simulink model "ev"  (R2021a)
settings: Solver=ode4  StartTime=0  StopTime=1082  FixedStep=sim_dt  RelTol=1e-3
model workspace (MAT data in the model file):
  T_eff_bp = [-270; -210; -150; -90; -30; 30; 90; 150; 210; 270]
  T_eff_bp_2 = [-270; -210; -150; -90; -30; 30; 90; 150; 210; 270]
  losses_table = [108927.107777 7820.2782368 7820.17609997 7820.2782368 7820.2782368 7820.2782368 7820.2782368 7820.26172359 7820.2782368 9345.38006027 108927.107777 7820.2782368 ... (100 elements, 10x10)]
  losses_table_2 = [108927.107777 7820.2782368 7820.17609997 7820.2782368 7820.2782368 7820.2782368 7820.2782368 7820.26172359 7820.2782368 9345.38006027 108927.107777 7820.2782368 ... (100 elements, 10x10)]
  w_eff_bp = [0; 888.888888889; 1777.77777778; 2666.66666667; 3555.55555556; 4444.44444444; 5333.33333333; 6222.22222222; 7111.11111111; 8000]
  w_eff_bp_2 = [0; 888.888888889; 1777.77777778; 2666.66666667; 3555.55555556; 4444.44444444; 5333.33333333; 6222.22222222; 7111.11111111; 8000]
undefined symbols (not defined in the file): Af, alpha, Bt, C, C_fa, C_free, C_sa_bat, C_sa_uc, Cd, Cmax, Continuous, Crr, DoD, effi, etaFD, etaG, FD, G, gear, Iucmax, m, M1m, M2m, Max, npar, npar_free, npara, nparf, nparfa, nparsa_bat, nparsa_UC, nser, nser_free, nserfa, nsersa_bat, nsersa_UC, Qbat, regenmax, Ri_BP, RL, ro, Rsc, Rsc_A, Rsc_F, Rsc_sa_bat, Rsc_sa_uc, rw, sim_dt, SOC_BP, SoCbatmax, SoCbatmin, SoCucmax, SoCucmin, speed, torque, VinBat, Voc_BP, Vuc, Vuc_fa, Vuc_free ... (+2)
libraries: autolibshared x41, simulink x26, autolibdcdc x13, autolibdatasheetbattery x7, autolibmappedmotor x6, fl_lib x3, nesl_utility x3, spsSupercapacitorLib x3, pid_lib x1
(part 3 of 18)

== system ev/Drive cycle power demand/Controller. Actual motor torque ==
  motor angular speed : Inport
  wheel torque : Inport  Port=2
  Power_motor_out : Inport  Port=3
  1-D Lookup Table : Lookup_n-D  NumberOfTableDimensions=1  BreakpointsForDimension1=Continuous(:,1)  Table=Continuous(:,2)  InternalRulePriority=Speed  RndMeth=Simplest  InputSameDT=on
  1-D Lookup Table2 : Lookup_n-D  NumberOfTableDimensions=1  BreakpointsForDimension1=Continuous(:,1)  Table=-Continuous(:,2)  InternalRulePriority=Speed  RndMeth=Simplest  InputSameDT=on
  Constant : Constant
  Delay : Delay  DelayLength=1  InitialCondition=1
  Delay1 : Delay  DelayLength=1  InitialCondition=0
  Equal : RelationalOperator  Operator===  OutDataTypeStr=boolean  RndMeth=Simplest
  Gain1 : Gain  Gain=30/pi
  Gain2 : Gain  Gain=30/pi
  Gain3 : Gain  Gain=30/pi
  GreaterThanOrEqual : RelationalOperator  OutDataTypeStr=boolean  RndMeth=Simplest
  MATLAB Function : MATLAB Function  TreatAsAtomicUnit=on
  Mux1 : Mux  Inputs=3
  Mux2 : Mux  Inputs=2
  Mux3 : Mux  Inputs=2
  Product : Product
  Product1 : Product
  Product2 : Product
  Saturation Dynamic : simulink/Discontinuities/Saturation Dynamic  OutMin=[]  OutMax=[]  OutDataTypeStr=Inherit: Same as second input  OutDataType=fixdt(1, 16)  OutScaling=2^-10  DoSatur=off
  Scope{6..14} (9 alike) : Scope
  Tapped Delay : simulink/Discrete/Tapped Delay  vinit=1  samptime=-1  NumDelays=30  DelayOrder=Oldest  includeCurrent=off
  To Workspace : ToWorkspace  VariableName=n_mtr  SaveFormat=Structure With Time  SampleTime=-1
  To Workspace1 : ToWorkspace  VariableName=com  SaveFormat=Structure With Time  SampleTime=-1
  To Workspace2 : ToWorkspace  VariableName=zz_motor_trq  SaveFormat=Structure With Time  SampleTime=-1
  To Workspace3 : ToWorkspace  VariableName=zz_motor_speed  SaveFormat=Structure With Time  SampleTime=-1
  To Workspace4 : ToWorkspace  VariableName=zz_gearshift  SaveFormat=Structure With Time  SampleTime=-1
  Motor power contr : Outport
  tag scope: gear_ratio=global, gear_shift=global, mtr_speed=global, mtr_trq=global, mtr_trq_corr=global
  wires:
  Power_motor_out/1 -> MATLAB Function/3(P_veh)
  wheel torque/1 -> Product/2, MATLAB Function/1(trq_wh)
  motor angular speed/1 -> Scope14/1, Product/1, MATLAB Function/2(w_wh)
  MATLAB Function/1(g1) -> [gear_ratio], Scope6/1
  MATLAB Function/2(Tau_def) -> Mux1/1, To Workspace2/1, [mtr_trq], Product1/1
  MATLAB Function/3(WG_def) -> Product1/2, Gain1/1, To Workspace3/1, [mtr_speed]
  Constant/1 -> MATLAB Function/4(g0)
  MATLAB Function/5(Tmax) -> Mux1/2
  MATLAB Function/6(Tmin) -> Mux1/3
  Mux1/1 -> Scope7/1
  [mtr_speed] -> Gain2/1, Product2/1
  [mtr_trq] -> Saturation Dynamic/2
  1-D Lookup Table/1 -> Saturation Dynamic/1
  1-D Lookup Table2/1 -> Saturation Dynamic/3
  Saturation Dynamic/1 -> Mux2/2, Product2/2, [mtr_trq_corr]
  [mtr_trq] -> Mux2/1
  Mux2/1 -> Scope10/1
  Product/1 -> Mux3/2
  Mux3/1 -> Scope11/1
  Product1/1 -> Mux3/1
  Product2/1 -> Motor power contr/1
  MATLAB Function/4(gs) -> To Workspace4/1, Scope9/1, [gear_shift]
  MATLAB Function/7(n_mtr) -> To Workspace/1
  Delay/1 -> Tapped Delay/1, Equal/1, MATLAB Function/5(g_prev)
  MATLAB Function/8(com) -> Scope12/1, To Workspace1/1
  Tapped Delay/1 -> Equal/2
  [gear_shift] -> Delay/1
  Equal/1 -> MATLAB Function/6(test)
  Gain1/1 -> Scope8/1
  Gain2/1 -> 1-D Lookup Table2/1, 1-D Lookup Table/1
  MATLAB Function/9(WG) -> Gain3/1
  Gain3/1 -> Scope13/1
  [vel_or] -> GreaterThanOrEqual/1, Delay1/1
  Delay1/1 -> GreaterThanOrEqual/2
  GreaterThanOrEqual/1 -> MATLAB Function/7(Vtest)
  [switch] -> MATLAB Function/8(mode)

== system ev/Drive cycle power demand/Motor torque estimation ==
  Force : Inport
  Constant : Constant  Value=FD
  Divide : Product  Inputs=*/
  Gain1 : Gain  Gain=rw
  Gain2 : Gain  Gain=1/etaFD
  Gain3 : Gain  Gain=etaFD
  Switch2 : Switch
  wheel torque : Outport
  tag scope: motor_trq=global, trq_wh=global
  wires:
  Divide/1 -> Gain2/1, Switch2/2, Gain3/1
  Gain2/1 -> Switch2/1  "motor_torque"
  Force/1 -> Gain1/1
  Constant/1 -> Divide/2
  Gain1/1 -> [trq_wh], wheel torque/1, Divide/1  "traction torque wheel"
  Gain3/1 -> Switch2/3  "breaking torque"
  Switch2/1 -> [motor_trq]  "motor torque output"

== system ev/Drive cycle power demand/Power estimation ==
  vel_m/s : Inport
  Force : Inport  Port=2
  Divide1 : Product  Inputs=*/
  Divide2 : Product  Inputs=**
  FD eff : Constant  Value=etaFD
  Product : Product
  Switch : Switch  Criteria=u2 > Threshold
  Terminator : Terminator
  To Workspace8 : ToWorkspace  VariableName=P_des  SaveFormat=Structure With Time  SampleTime=-1
  Power_motor_out : Outport
  tag scope: P_veh=global
  wires:
  vel_m/s/1 -> Product/1
  Product/1 -> Power_motor_out/1, To Workspace8/1, Switch/2, Divide2/1, Divide1/1, [P_veh]  "traction power"
  Divide1/1 -> Switch/1  "motor power"
  FD eff/1 -> Divide2/2, Divide1/2
  Divide2/1 -> Switch/3  "Braking_power"
  Force/1 -> Product/2
  Switch/1 -> Terminator/1  "Power_motor"

== system ev/Drive cycle power demand/Veh force estimation ==
  vel_m/s : Inport
  Acceleration : Inport  Port=2
  0.01 : Constant  Value=Crr
  0.1 : Constant  Value=3.6
  0.2 : Constant  Value=100
  A : Product  Inputs=*/
  Add : Sum
  Aerodynamic_drag : Subsystem
  B : Constant
  Constant : Constant  Value=9.81
  Constant1 : Constant  Value=sim_dt
  Delay5 : Delay  DelayLength=1  InitialCondition=0
  Derivative : Derivative  CoefficientInTFapproximation=0.001
  Distance travelled : DisplayBlock  LabelPosition=Hide  Format=shortEng  Transparency=1
  Divide1 : Product  Inputs=*/
  Gain4 : Gain
  Hill_climbing_force : Subsystem
  Integrator : Integrator
  Linear_acceleration : Subsystem
  Manual Switch : ManualSwitch  CurrentSetting=0
  Mux : Mux  Inputs=3
  Product2 : Product
  Rolling resistance : Subsystem
  Scope{,1..5,12} (7 alike) : Scope
  Subtract : Sum  Inputs=+-
  Sum : Sum  Inputs=++++
  To Workspace : ToWorkspace  VariableName=Fad  SaveFormat=Structure With Time  SampleTime=-1
  To Workspace1 : ToWorkspace  VariableName=Fhc  SaveFormat=Structure With Time  SampleTime=-1
  To Workspace2 : ToWorkspace  VariableName=Ft  SaveFormat=Structure With Time  SampleTime=-1
  To Workspace5 : ToWorkspace  VariableName=Fa  SaveFormat=Structure With Time  SampleTime=-1
  To Workspace6 : ToWorkspace  VariableName=Frr  SaveFormat=Structure With Time  SampleTime=-1
  air density : Constant  Value=ro
  drag coefficient : Constant  Value=Cd
  frontal area : Constant  Value=Af
  rolling resistance coefficient : Product
  vehicle mass : Constant  Value=m
  Total force : Outport
  tag scope: F_ad=global, F_hc=global, F_la=global, F_rr=global, F_veh=global
  wires:
  frontal area/1 -> Aerodynamic_drag/3(frontal_area)
  Rolling resistance/1(Fhc) -> To Workspace6/1, Scope2/1, [F_rr], Sum/4
  Aerodynamic_drag/1(Fad) -> To Workspace/1, Scope5/1, [F_ad], Sum/1
  [deg] -> Rolling resistance/4(theta), Hill_climbing_force/4(Theta)
  Linear_acceleration/1(Fhc) -> To Workspace5/1, Scope3/1, [F_la], Gain4/1
  air density/1 -> Aerodynamic_drag/2(air_density)
  Sum/1 -> [F_veh], Scope/1, Total force/1, To Workspace2/1  "Total force"
  Hill_climbing_force/1(Fhc) -> To Workspace1/1, [F_hc], Scope4/1, Sum/2
  Gain4/1 -> Sum/3
  0.1/1 -> A/1
  A/1 -> Product2/2
  B/1 -> Add/2
  Product2/1 -> Add/1
  Add/1 -> rolling resistance coefficient/2
  vehicle mass/1 -> Rolling resistance/1(vehicle_mass), Linear_acceleration/2(Veh_mass), Hill_climbing_force/2(vehicle_mass)
  Constant/1 -> Rolling resistance/3(gravity), Hill_climbing_force/3(Gravity)
  0.01/1 -> Manual Switch/1, rolling resistance coefficient/1
  0.2/1 -> A/2
  drag coefficient/1 -> Aerodynamic_drag/4(Drag_coefficient)
  Integrator/1 -> Scope12/1  "distance travelled m"
  vel_m/s/1 -> Delay5/1, Subtract/1, Aerodynamic_drag/1(vel_m/s), Hill_climbing_force/1(vel_m/s), Derivative/1, Integrator/1, Rolling resistance/5(v m/s), Product2/1  "vel m/s"
  Acceleration/1 -> Mux/3, Linear_acceleration/1(Acceleration)
  Mux/1 -> Scope1/1
  Derivative/1 -> Mux/1
  Manual Switch/1 -> Rolling resistance/2(Rolling_resistance)
  rolling resistance coefficient/1 -> Manual Switch/2
  Delay5/1 -> Subtract/2
  Subtract/1 -> Divide1/1
  Constant1/1 -> Divide1/2
  Divide1/1 -> Mux/2

== system ev/Drive cycle power demand/motor speed estimation ==
  vel_m/s : Inport
  Constant : Constant  Value=FD
  Gain : Gain  Gain=1/(rw)
  Scope1 : Scope
  To Workspace3 : ToWorkspace  VariableName=w  SaveFormat=Structure With Time  SampleTime=-1
  gear shift : Constant  Commented=on  Value=gear
  transmission : Product
  motor angular speed rad/s : Outport
  tag scope: w_wh=global
  wires:
  transmission/1 -> To Workspace3/1, Scope1/1  "motor angular speed"
  Constant/1 -> transmission/2
  Gain/1 -> motor angular speed rad/s/1, [w_wh], transmission/1  "wheel angular speed"
  vel_m/s/1 -> Gain/1

== system ev/Seleccion de ciclo de manejo/Subsystem ==
  Vel_m/s : Inport
  Acel @vel const : Inport  Port=2
  Constant1 : Constant  Value=sim_dt
  Delay5 : Delay  DelayLength=1  InitialCondition=0
  Derivative : Derivative  CoefficientInTFapproximation=0.001
  Divide1 : Product  Inputs=*/
  Mux : Mux  Inputs=3
  Scope1 : Scope
  Scope2 : Scope
  Subtract : Sum  Inputs=+-
  Vel : Outport
  Accel : Outport  Port=2
  wires:
  Derivative/1 -> Mux/1, Accel/1
  Subtract/1 -> Divide1/1
  Delay5/1 -> Subtract/2
  Vel_m/s/1 -> Derivative/1, Delay5/1, Subtract/1, Vel/1, Scope2/1
  Mux/1 -> Scope1/1
  Constant1/1 -> Divide1/2
  Divide1/1 -> Mux/2
  Acel @vel const/1 -> Mux/3

== system ev/Seleccion de ciclo de manejo/Velocity ==
  vel_km/h : Inport
  Gain : Gain  Gain=1/3.6
  Integrator : Integrator
  Scope : Scope
  To Workspace : ToWorkspace  VariableName=dist_m  SaveFormat=Timeseries  SampleTime=-1
  Vel_m/s : Outport  VectorParamsAs1DForOutWhenUnconnected=off
  wires:
  Integrator/1 -> To Workspace/1, Scope/1  "dist_meters"
  Gain/1 -> Vel_m/s/1, Integrator/1
  vel_km/h/1 -> Gain/1

== system ev/Seleccion de ciclo de manejo/Velocity1 ==
  vel_km/h : Inport
  Gain : Gain  Gain=1/3.6
  Integrator : Integrator
  Scope : Scope
  Scope2 : Scope
  Vel_m/s : Outport  VectorParamsAs1DForOutWhenUnconnected=off
  wires:
  Integrator/1 -> Scope/1  "dist_meters"
  Gain/1 -> Vel_m/s/1, Integrator/1
  vel_km/h/1 -> Scope2/1, Gain/1

== system ev/Subsystem/motor speed estimation ==
  vel_m/s : Inport
  Gain : Gain  Gain=1/(rw)
  Scope1 : Scope
  transmission : Product
  motor angular speed : Outport
  wires:
  transmission/1 -> motor angular speed/1, Scope1/1  "motor angular speed"
  [gear_ratio] -> transmission/2
  Gain/1 -> transmission/1  "wheel angular speed"
  vel_m/s/1 -> Gain/1

== system ev/Tesis/Battery model ==
  motor_pwr_contr : Inport
  Add : Sum  Inputs=+-
  Bus Selector : BusSelector  OutputSignals=BattSoc,BattCurr,BattPwr,BattAmpHr
  Constant2 : Constant  Value=293.15
  Current_calc : Product  Inputs=/*
  Datasheet Battery : autolibdatasheetbattery/Datasheet Battery  CapacityCtrl=Parameter  OutputVlt=Unfiltered  BattChargeMax=Qbat  Em=Voc_BP  CapLUTBp=SOC_BP  RInt=iR_bp  BattTempBp=Temp_bp  CapSOCBp=SOC_BP  Ns=nser  Np=npar  BattCapInit=Qbat*(1-DoD)  Tc=0.01  Vinit=3.3342*nser  RefBlkName='autolibdatasheetbattery/Datasheet Battery'
      settings: SourceProductBaseCode=PW
  Display1 : DisplayBlock  LabelPosition=Hide  Format=short  Transparency=1
  Gain4 : Gain  Gain=nser
  Gain5 : Gain  Gain=nser/npar
  MATLAB Function1 : MATLAB Function  TreatAsAtomicUnit=on
  Mux : Mux
  Mux12 : Mux  Inputs=2
  OCV1 : Lookup_n-D  NumberOfTableDimensions=1  BreakpointsForDimension1=SOC_BP  Table=Voc_BP  InternalRulePriority=Speed  RndMeth=Simplest  InputSameDT=on
  Product : Product
  Product1 : Product
  Ri1 : Lookup_n-D  NumberOfTableDimensions=1  BreakpointsForDimension1=SOC_BP  Table=Ri_BP  InternalRulePriority=Speed  RndMeth=Simplest  InputSameDT=on
  Scope{1..2,6..7,13..14,26,39,44} (9 alike) : Scope
  Subsystem : Subsystem
  To Workspace9 : ToWorkspace  VariableName=Batt  SaveFormat=Structure With Time  SampleTime=-1
  vehicle dynamics : Subsystem
  tag scope: block=global
  wires:
  Bus Selector/2 -> Scope26/1, Product1/2  "<BattCurr>"
  Gain5/1 -> MATLAB Function1/1(Ri), Product1/1, Scope1/1
  Datasheet Battery/2 -> Product/2, Mux/2  "Voltage"
  Bus Selector/1 -> [block], Scope7/1, Ri1/1, OCV1/1  "<BattSoc>"
  Mux/1 -> Scope14/1
  Gain4/1 -> Add/1, Mux/1, Current_calc/1
  OCV1/1 -> Gain4/1
  Bus Selector/3 -> Subsystem/1(power), Mux12/1  "<BattPwr>"
  Ri1/1 -> Gain5/1
  Add/1 -> Mux/3
  MATLAB Function1/1(Vb) -> Mux/4, Scope44/1
  Product1/1 -> Add/2
  Mux12/1 -> Scope39/1
  Datasheet Battery/1 -> Scope6/1, Bus Selector/1, To Workspace9/1
  Constant2/1 -> Datasheet Battery/2
  Current_calc/1 -> MATLAB Function1/2(Ib), Datasheet Battery/1, Scope13/1  "I_batt"
  motor_pwr_contr/1 -> Mux12/2, Subsystem/2(motor_pwr_contr), MATLAB Function1/3(Pmot), Current_calc/2
  Subsystem/1(Out1) -> vehicle dynamics/1("Force_FA ")
  Bus Selector/4 -> Product/1  "<BattAmpHr>"
  Product/1 -> Scope2/1  "Wh"
